simulink model "SimulinkEnv"  (R2024a)
settings: Solver=FixedStepAuto  StartTime=0.0  StopTime=2  RelTol=1e-3
model workspace (MAT data in the model file):
  SL_ROS_VariableLengthArrays_MaxSizes.CommonInfo.ArrayTruncateAction = 'EmitWarning'
  SL_ROS_VariableLengthArrays_MaxSizes.MsgTypeMap = containers.Map
  SL_ROS_VariableLengthArrays_MaxSizes.MsgTypeMap.serialization.keys = {'sensor_msgs/Image'}
  SL_ROS_VariableLengthArrays_MaxSizes.MsgTypeMap.serialization.values{1}(1).PropertyName = 'data'
  SL_ROS_VariableLengthArrays_MaxSizes.MsgTypeMap.serialization.values{1}(1).DataType = 'uint8'
  SL_ROS_VariableLengthArrays_MaxSizes.MsgTypeMap.serialization.values{1}(1).MaxLength = 2764800
  SL_ROS_VariableLengthArrays_MaxSizes.MsgTypeMap.serialization.values{1}(2).PropertyName = 'encoding'
  SL_ROS_VariableLengthArrays_MaxSizes.MsgTypeMap.serialization.values{1}(2).DataType = 'uint8'
  SL_ROS_VariableLengthArrays_MaxSizes.MsgTypeMap.serialization.values{1}(2).MaxLength = 128
  SL_ROS_VariableLengthArrays_MaxSizes.MsgTypeMap.serialization.uniformity = 0
  SL_ROS_VariableLengthArrays_MaxSizes.MsgTypeMap.serialization.keyType = 'char'
  SL_ROS_VariableLengthArrays_MaxSizes.MsgTypeMap.serialization.valueType = 'any'
undefined symbols (not defined in the file): approx_tag_length_cm, Box_pos, BX_x, BX_y, BX_z, coder, home_pos, P_x, P_y, P_z, ros, rTagLocs, Sim3dSensor, SP_pos, stewart_config
libraries: sim3dlib x21, ros2lib x2, sim3dcameralib x2, uavsim3dlib x2, simulink_extras x1, dspvision x1, visionsinks x1, simulink x1
settings Model: PauseTimes=0.5  Creator=dylanfanner  LastModifiedBy=alyss
settings OptimizationCC: EnhancedBackFolding=on  PassReuseOutputArgsAs=Individual arguments  ZeroExternalMemoryAtStartup=off  ZeroInternalMemoryAtStartup=off  MaxStackSize=64  OptimizeBlockOrder=speed  DifferentSizesBufferReuse=on  OptimizationCustomize=off  EfficientTunableParamExpr=on
settings DebuggingCC: ParameterTunabilityLossMsg=error
settings HardwareCC: ProdBitPerLong=64  ProdHWDeviceType=Intel->x86-64 (Linux 64)
settings SFSimCC: MATLABDynamicMemAlloc=off
settings RTWCC: Description=Embedded Coder  SystemTargetFile=ert.tlc  HardwareBoard=Robot Operating System 2 (ROS 2)  TLCOptions="-aInlineSetEventsForThisBaseRateFcn=TLC_FALSE -aSuppressMultiTaskScheduler=TLC_FALSE  -aRateBasedStepFcn=0"  TemplateMakefile=ert_default_tmf  Toolchain=Colcon Tools  TargetLang=C++
settings CodeAppCC: ForceParamTrailComments=on  IgnoreCustomStorageClasses=off  OperatorAnnotations=on  SimulinkDataObjDesc=on  SFDataObjDesc=on  InsertBlockDesc=on
settings ERTTargetCC: CodeInterfacePackaging=C++ class  RootIOFormat=Structure reference

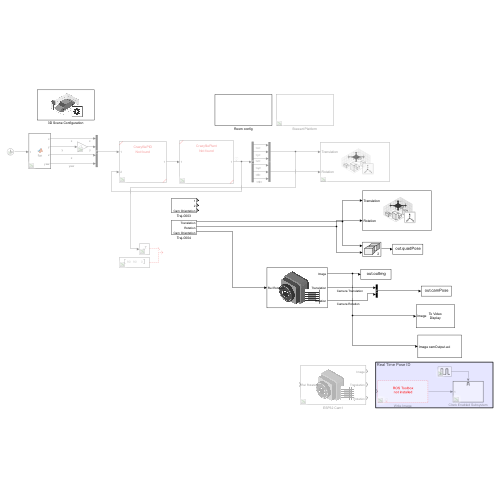
[thumbnail: Simulink's stored preview of the top-level diagram]
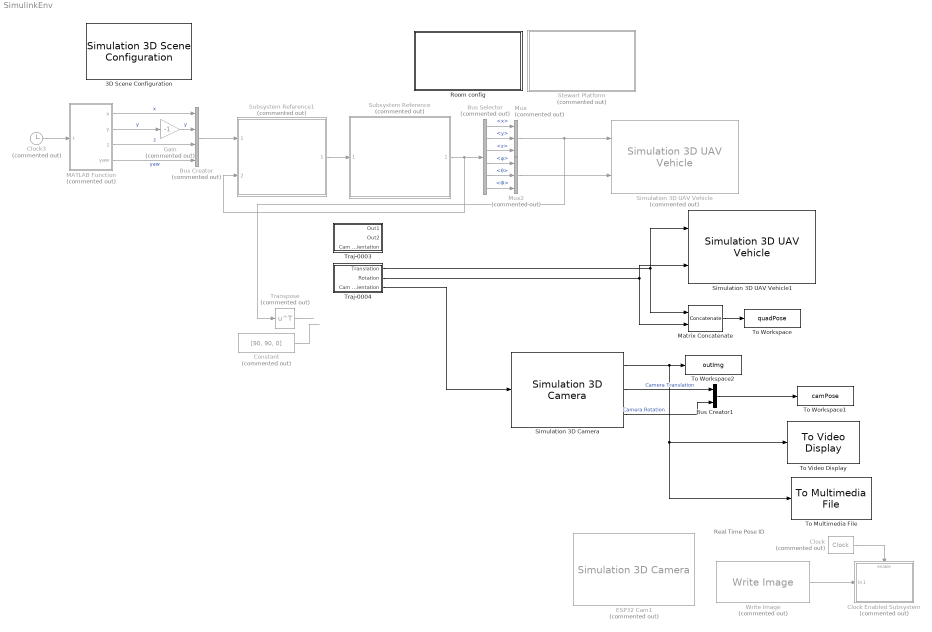
== system SimulinkEnv ==
  note: Real Time Pose ID
  3D Scene Configuration : sim3dlib/Simulation 3D Scene Configuration  Priority=0  ProjectFormat=Default Scenes  SceneDesc=Empty scene  ProjectName=C:\Programs\MATLAB\R2024a\toolbox\shared\sim3d_projects\automotive_project_windows\UE\WindowsNoEditor\VehicleSimulation.exe  ScenePath=/Game/Maps/HwStrght  EnableOpenDRIVE=off  vehTagList={'CrazyFlie';'Custom';'GenericQuad1';'Scene Origin';'Sim3dActor3'}  vehTag=Scene Origin  FreeCameraInitialTranslation=[0, 0, 0]  FreeCameraDefaultInitialTranslation=[-6, 0, 2]  FreeCameraInitialRotation=[0, 0, 0]  FreeCameraDefaultInitialRotation=[0, -15, 0]  OpVisEn=off  Ts=.01  EnableWindow=on  EnableRemoteAccess=off  EnableWeather=off  SunAzimuth=90  SunAltitude=40.0  EnableGeospatialSun=off  Latitude=0  Longitude=0  Date=2023-01-01  Time=10:30:00  GeoTimeZone=-5.0  SunDaylightSaving=off  wind=1  clouds=10  EnableVolumetricClouds=off  CloudCoverage=0  CloudAltitude=6  fog=0  rain=0  RaindropsEffect=off  SnowDensity=0.0  EnableGeospatial=off  UseTrueOrigin=off  OriginHeight=200  OriginLatitude=40.744652  OriginLongitude=-73.988864  MapStyle=Aerial  AdditionalAssetIDs=[]  UseAdvancedSunSky=off  SolarTime=11  TimeZone=-5  Day=21  Month=9  Year=2022  UseDaylightSavingTime=on  DSTStartDay=10  DSTStartMonth=3  DSTEndDay=3  DSTEndMonth=11  DSTSwitchHour=2  sensorTag=MainCamera1  sensorId=1  sensorName=MainCamera1  mountLoc=Origin  offsetFlag=off  tmountOffset=[0, 0, 0]  rmountOffset=[0, 0, 0]  HorizontalResolution=1280  VerticalResolution=720  HorizontalFOV=60  mountPoint=[0 0 0]  mountOrientation=[0 0 0]  aMode=5  ID=1  GeoTrigger=Inactive
      settings: LibrarySourceBlock=sl3dlib/Simulation 3D/Environment/Simulation 3D Scene Configuration
  Bus Creator : BusCreator  Commented=on  Inputs=4
  Bus Creator1 : BusCreator  Inputs=2
  Bus Selector : BusSelector  Commented=on  OutputSignals=Position State.position.x,Position State.position.y,Position State.position.z,Attitude State.attitude.ψ,Attitude State.attitude.θ,Attitude State.attitude.Φ
  Clock : simulink_extras/Flip Flops/Clock  Commented=on  period=0.25
  Clock Enabled Subsystem : Subsystem  Commented=on
  Clock3 : Clock  Commented=on
  Constant : Constant  Commented=on  Value=[90, 90, 0]  VectorParams1D=off
  ESP32 Cam1 : sim3dcameralib/Simulation 3D Camera  Priority=1  Commented=on  sensorTag=Sim3dSensor�  sensorId=3  sensorName=Sim3dSensor�  vehTagList={'CrazyFlie';'Floor';'SPBox';'SPP';'SPapriltexture';'Scene Origin';'Wall1';'Wall2'}  vehTag=CrazyFlie  mountLoc=Origin  offsetFlag=on  tmountOffset=[0, 0, 0]  extTmount=off  rmountOffset=[0, 0, 0]  extRmount=on  FocalLength=cameraParams.FocalLength  OpticalCenter=[640, 360] % I think this is fine  ImageSize=cameraParams.ImageSize  RadialDistortion=cameraParams.RadialDistortion  TangentialDistortion=cameraParams.TangentialDistortion  SensorSkew=0  DepthOutportEnabled=off  SemanticOutportEnabled=off  TransformOutportEnabled=on  SampleTime=-1  mountPoint=[0 0 0]  mountOrientation=[0 0 0]  aMode=6  ID=3
      settings: LibrarySourceBlock=robotsim3dlib/Simulation 3D Camera
  Gain : Gain  Commented=on  Gain=-1
  MATLAB Function : MATLAB Function  Commented=on  TreatAsAtomicUnit=on
  Matrix Concatenate : Concatenate  Mode=Multidimensional array  ConcatenateDimension=2
  Mux : Mux  Commented=on  Inputs=3
  Mux2 : Mux  Commented=on  Inputs=3
  Room config : Subsystem
  Simulation 3D Camera : sim3dcameralib/Simulation 3D Camera  Priority=1  sensorTag=Sim3dSensor�  sensorId=2  sensorName=Sim3dSensor�  vehTagList={'CrazyFlie';'GenericQuad1';'Scene Origin';'Sim3dActor3'}  vehTag=GenericQuad1  mountLoc=Origin  offsetFlag=on  tmountOffset=[0, 0, 0]  extTmount=off  rmountOffset=[0, 0, 0]  extRmount=on  FocalLength=[1107, 1107]  OpticalCenter=[640, 360]  ImageSize=[720, 1280]  RadialDistortion=[0, 0]  TangentialDistortion=[0, 0]  SensorSkew=0  DepthOutportEnabled=off  SemanticOutportEnabled=off  TransformOutportEnabled=on  SampleTime=1/10  mountPoint=[0 0 0]  mountOrientation=[0 0 0]  aMode=6  ID=2
      settings: LibrarySourceBlock=robotsim3dlib/Simulation 3D Camera
  Simulation 3D UAV Vehicle : uavsim3dlib/Simulation 3D UAV Vehicle  Priority=-1  Commented=on  Mesh=Quadrotor  MeshPath=/MathWorksUAVContent/UAVs/HexaRotorUAV/HexaRotor.HexaRotor  Color=Black  ActorName=CrazyFlie  UseGlobalFrame=off  InitialTranslation=[0 0 0]  InitialRotation=[0 0 0]  InitialTranslationGlobal=[0 0 0]  InitialGeoOrigin=[0 0 0]  InitialRotationGlobal=[0 0 0]  SampleTime=-1  ActorType=SimulinkVehicle  ID=C  aMode=4  ActorTag=CrazyFlie
  Simulation 3D UAV Vehicle1 : uavsim3dlib/Simulation 3D UAV Vehicle  Priority=-1  Mesh=Quadrotor  MeshPath=/MathWorksUAVContent/UAVs/HexaRotorUAV/HexaRotor.HexaRotor  Color=Black  ActorName=GenericQuad1  UseGlobalFrame=off  InitialTranslation=[-3 0 1]  InitialRotation=[0 0 0]  InitialTranslationGlobal=[0 0 0]  InitialGeoOrigin=[0 0 0]  InitialRotationGlobal=[0 0 0]  SampleTime=-1  ActorType=SimulinkVehicle  ID=C  aMode=4  ActorTag=GenericQuad1
  Stewart Platform : Subsystem  Commented=on
  Subsystem Reference : Subsystem  Commented=on  ReferencedSubsystem=CrazyfliePlant
  Subsystem Reference1 : Subsystem  Commented=on  ReferencedSubsystem=CrazyfliePID
  To Multimedia File : dspvision/To Multimedia File  outputFilename=camOutput.avi  streamSelection=Video only  videoCompressor=None (uncompressed)  audioCompressor=None (uncompressed)  imagePorts=One multidimensional signal  fileType=AVI  audioDatatype=Determine from input data type  fourcc=RGB  audioBitRate=128  audioQuality=75  videoQuality=75  mj2000CompFactor=10
      settings: LibrarySourceBlock=visionsinks/To Multimedia File
  To Video Display : visionsinks/To Video Display  windowSizeMode=Normal  openAtMdlStart=on  fullScreen=off  videoWindowX=0  videoWindowY=23  saveWindowSize=off  videoWindowWidth=1366  videoWindowHeight=745  inputColorFormat=RGB  inputType=Obsolete  imagePorts=One multidimensional signal  OutputDevice=On-screen video monitor  dataOrg=Column-major  isWindowOpen=off
  To Workspace : ToWorkspace  VariableName=quadPose  SaveFormat=Structure With Time  SampleTime=0.1
  To Workspace1 : ToWorkspace  VariableName=camPose  SaveFormat=Structure With Time  SampleTime=0.1
  To Workspace2 : ToWorkspace  VariableName=outImg  SaveFormat=Structure With Time  SampleTime=0.1
  Traj-0003 : Subsystem
  Traj-0004 : Subsystem
  Transpose : Math  Commented=on  Operator=transpose
  Write Image : ros2lib/Write Image  Commented=on  ImageEncoding=rgb8  EncodingStruct=ros.msg.sensor_msgs.internal.ImageEncoding.info(coder.const('rgb8'))  HasAlpha=off  messageType=sensor_msgs/Image
  wires:
  Subsystem Reference1/1 -> Subsystem Reference/1
  Subsystem Reference/1 -> Subsystem Reference1/2, Bus Selector/1
  Bus Selector/2 -> Mux/2  "<y>"
  Bus Selector/3 -> Mux/3  "<z>"
  Bus Selector/1 -> Mux/1  "<x>"
  Bus Selector/5 -> Mux2/2  "<θ>"
  Bus Selector/4 -> Mux2/1  "<ψ>"
  Bus Selector/6 -> Mux2/3  "<Φ>"
  Bus Creator/1 -> Subsystem Reference1/1
  MATLAB Function/3(z) -> Bus Creator/3  "z"
  MATLAB Function/4(yaw) -> Bus Creator/4  "yaw"
  Mux2/1 -> Simulation 3D UAV Vehicle/2
  Simulation 3D Camera/1 -> To Video Display/1, To Multimedia File/1, To Workspace2/1
  Simulation 3D Camera/3 -> Bus Creator1/2  "Camera Rotation"
  Simulation 3D Camera/2 -> Bus Creator1/1  "Camera Translation"
  Write Image/1 -> Clock Enabled Subsystem/1(In1)
  Clock/1 -> Clock Enabled Subsystem/Enable
  Bus Creator1/1 -> To Workspace1/1
  Gain/1 -> Bus Creator/2  "y"
  Mux/1 -> Simulation 3D UAV Vehicle/1, Transpose/1
  MATLAB Function/1(x) -> Bus Creator/1  "x"
  MATLAB Function/2(y) -> Gain/1  "y"
  Clock3/1 -> MATLAB Function/1(t)
  Constant/1 -> ?
  Transpose/1 -> ?
  Matrix Concatenate/1 -> To Workspace/1
  Traj-0004/1(Translation) -> Simulation 3D UAV Vehicle1/1, Matrix Concatenate/1
  Traj-0004/2(Rotation) -> Simulation 3D UAV Vehicle1/2, Matrix Concatenate/2
  Traj-0004/3(Cam Orientation) -> Simulation 3D Camera/1

== system SimulinkEnv/Clock Enabled Subsystem ==
  In1 : Inport
  Enable : EnablePort
  Publish : ros2lib/Publish  topicSource=Specify your own  topic=/simCam/imgOut  messageType=sensor_msgs/Image  QOSHistory=Keep last  QOSDepth=1  QOSReliability=Reliable  QOSDurability=Volatile  QOSDeadline=Inf  QOSLifespan=Inf  QOSLiveliness=Automatic  QOSLeaseDuration=Inf  QOSAvoidROSNamespaceConventions=off
  wires:
  In1/1 -> Publish/1

== system SimulinkEnv/Room config ==
  Apriltags : sim3dlib/Simulation 3D Actor  Priority=1  ActorName=Sim3dActor1  ParentName=Scene Origin  Operation=Create at setup  InitScriptText=|  SampleTime=-1  Translation=single([0 0 0])  Rotation=single([0 0 0])  Scale=single([1 1 1])  aMode=5  ActorTag=Sim3dActor1  ActorType=Sim3dActor  ID=1
      | % Reserved keywords:
      | % - Actor : handle to this actor object
      | % - World : handle to the world object
      | 
      | % Examples:
      | 
      | % Create a primitive geometry (optional)
      | % Actor.createShape('box', [1 1 1]);
      | 
      | % Initialize values (optional)
      | % Actor.Scale = 1;
      | % Actor.Color = [1 0 0];
  Checkerboards : sim3dlib/Simulation 3D Actor  Priority=1  ActorName=Sim3dActor2  ParentName=Scene Origin  Operation=Create at setup  InitScriptText=|  SampleTime=-1  Translation=single([0 0 0])  Rotation=single([0 0 0])  Scale=single([1 1 1])  aMode=5  ActorTag=Sim3dActor2  ActorType=Sim3dActor  ID=2
      | % Reserved keywords:
      | % - Actor : handle to this actor object
      | % - World : handle to the world object
      | 
      | % Examples:
      | 
      | % Create a primitive geometry (optional)
      | % Actor.createShape('box', [1 1 1]);
      | 
      | % Initialize values (optional)
      | % Actor.Scale = 1;
      | % Actor.Color = [1 0 0];
  Floor : sim3dlib/Simulation 3D Actor  Priority=1  ActorName=Sim3dActor3  ParentName=Scene Origin  Operation=Create at setup  InitScriptText=|  SampleTime=-1  Translation=single([0 0 0])  Rotation=single([0 0 0])  Scale=single([1 1 1])  aMode=5  ActorTag=Sim3dActor3  ActorType=Sim3dActor  ID=3
      | % Reserved keywords:
      | % - Actor : handle to this actor object
      | % - World : handle to the world object
      | 
      | % Examples:
      | 
      | % Create a primitive geometry (optional)
      | % Actor.createShape('box', [1 1 1]);
      | 
      | % Initialize values (optional)
      | % Actor.Scale = 1;
      | % Actor.Color = [1 0 0];
  Walls : sim3dlib/Simulation 3D Actor  Priority=1  ActorName=Sim3dActor4  ParentName=Scene Origin  Operation=Create at setup  InitScriptText=|  SampleTime=-1  Translation=single([0 0 0])  Rotation=single([0 0 0])  Scale=single([1 1 1])  aMode=5  ActorTag=Sim3dActor4  ActorType=Sim3dActor  ID=4
      | % Reserved keywords:
      | % - Actor : handle to this actor object
      | % - World : handle to the world object
      | 
      | % Examples:
      | 
      | % Create a primitive geometry (optional)
      | % Actor.createShape('box', [1 1 1]);
      | 
      | % Initialize values (optional)
      | % Actor.Scale = 1;
      | % Actor.Color = [1 0 0];

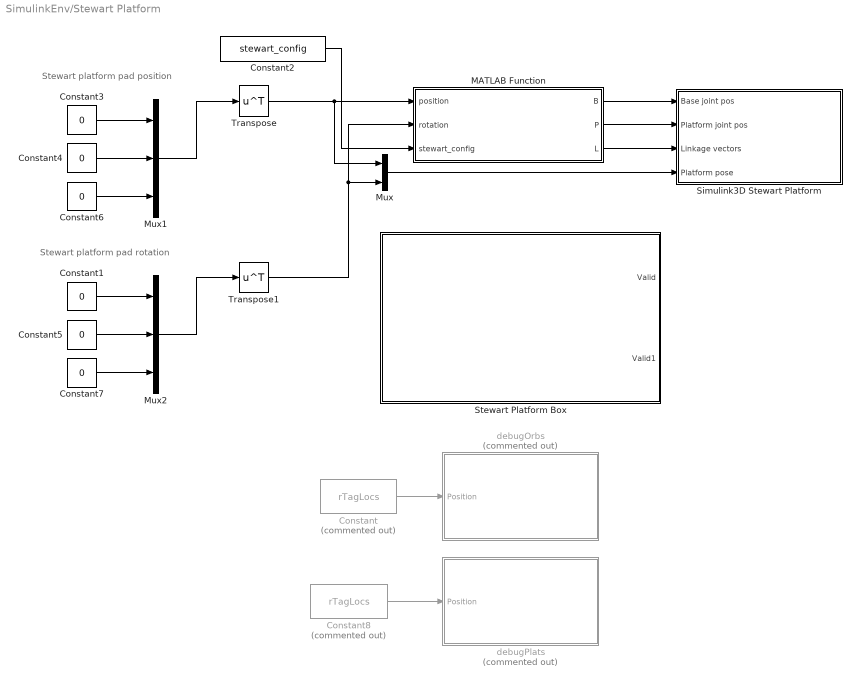
== system SimulinkEnv/Stewart Platform ==
  note: Stewart platform pad rotation
  note: Stewart platform pad position
  Constant : Constant  Commented=on  Value=rTagLocs
  Constant{1,3..7} (6 alike) : Constant  Value=0
  Constant2 : Constant  Value=stewart_config  VectorParams1D=off
  Constant8 : Constant  Commented=on  Value=rTagLocs
  MATLAB Function : MATLAB Function  TreatAsAtomicUnit=on
  Mux : Mux  Inputs=2
  Mux1 : Mux  Inputs=3
  Mux2 : Mux  Inputs=3
  Simulink3D Stewart Platform : Subsystem
  Stewart Platform Box : Subsystem
  Transpose : Math  Operator=transpose
  Transpose1 : Math  Operator=transpose
  debugOrbs : Subsystem  Commented=on  TreatAsAtomicUnit=on
  debugPlats : Subsystem  Commented=on  TreatAsAtomicUnit=on
  wires:
  Mux2/1 -> Transpose1/1
  MATLAB Function/2(P) -> Simulink3D Stewart Platform/2(Platform joint pos)
  Constant3/1 -> Mux1/1
  Constant4/1 -> Mux1/2
  Constant2/1 -> MATLAB Function/3(stewart_config)
  Constant5/1 -> Mux2/2
  Constant1/1 -> Mux2/1
  Mux1/1 -> Transpose/1
  Constant7/1 -> Mux2/3
  Mux/1 -> Simulink3D Stewart Platform/4(Platform pose)
  MATLAB Function/3(L) -> Simulink3D Stewart Platform/3(Linkage vectors)
  Constant6/1 -> Mux1/3
  Transpose1/1 -> MATLAB Function/2(rotation), Mux/2
  MATLAB Function/1(B) -> Simulink3D Stewart Platform/1(Base joint pos)
  Transpose/1 -> MATLAB Function/1(position), Mux/1
  Constant/1 -> debugOrbs/1(Position)
  Constant8/1 -> debugPlats/1(Position)

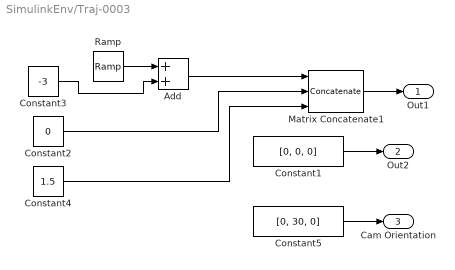
== system SimulinkEnv/Traj-0003 ==
  Add : Sum
  Constant1 : Constant  Value=[0, 0, 0]  VectorParams1D=off
  Constant2 : Constant  Value=0
  Constant3 : Constant  Value=-3
  Constant4 : Constant  Value=1.5
  Constant5 : Constant  Value=[0, 30, 0]  VectorParams1D=off
  Matrix Concatenate1 : Concatenate  NumInputs=3  Mode=Multidimensional array  ConcatenateDimension=2
  Ramp : simulink/Sources/Ramp  slope=0.5  start=0.2  InitialOutput=0
  Out1 : Outport
  Out2 : Outport  Port=2
  Cam Orientation : Outport  Port=3
  wires:
  Constant3/1 -> Add/2
  Ramp/1 -> Add/1
  Matrix Concatenate1/1 -> Out1/1
  Add/1 -> Matrix Concatenate1/1
  Constant1/1 -> Out2/1
  Constant2/1 -> Matrix Concatenate1/2
  Constant4/1 -> Matrix Concatenate1/3
  Constant5/1 -> Cam Orientation/1

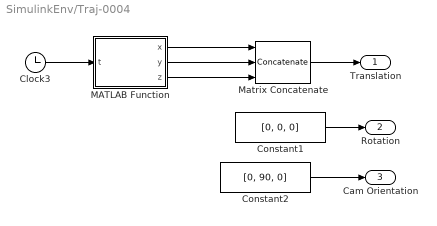
== system SimulinkEnv/Traj-0004 ==
  Clock3 : Clock
  Constant1 : Constant  Value=[0, 0, 0]  VectorParams1D=off
  Constant2 : Constant  Value=[0, 90, 0]  VectorParams1D=off
  MATLAB Function : MATLAB Function  TreatAsAtomicUnit=on
  Matrix Concatenate : Concatenate  NumInputs=3  Mode=Multidimensional array  ConcatenateDimension=2
  Translation : Outport
  Rotation : Outport  Port=2
  Cam Orientation : Outport  Port=3
  wires:
  Clock3/1 -> MATLAB Function/1(t)
  MATLAB Function/2(y) -> Matrix Concatenate/2
  MATLAB Function/3(z) -> Matrix Concatenate/3
  Matrix Concatenate/1 -> Translation/1
  MATLAB Function/1(x) -> Matrix Concatenate/1
  Constant1/1 -> Rotation/1
  Constant2/1 -> Cam Orientation/1

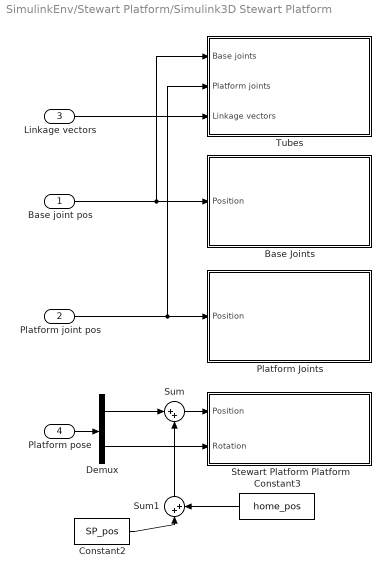
== system SimulinkEnv/Stewart Platform/Simulink3D Stewart Platform ==
  Base joint pos : Inport
  Platform joint pos : Inport  Port=2
  Linkage vectors : Inport  Port=3
  Platform pose : Inport  Port=4
  Base Joints : Subsystem  TreatAsAtomicUnit=on
  Constant2 : Constant  Value=SP_pos  VectorParams1D=off
  Constant3 : Constant  Value=home_pos  VectorParams1D=off
  Demux : Demux  Outputs=2
  Platform Joints : Subsystem  TreatAsAtomicUnit=on
  Stewart Platform Platform : Subsystem
  Sum : Sum  Inputs=|++
  Sum1 : Sum  Inputs=|++
  Tubes : Subsystem  TreatAsAtomicUnit=on
  wires:
  Base joint pos/1 -> Base Joints/1(Position), Tubes/1(Base joints)
  Platform joint pos/1 -> Platform Joints/1(Position), Tubes/2(Platform joints)
  Linkage vectors/1 -> Tubes/3(Linkage vectors)
  Demux/2 -> Stewart Platform Platform/2(Rotation)
  Platform pose/1 -> Demux/1
  Constant3/1 -> Sum1/2
  Constant2/1 -> Sum1/1
  Sum1/1 -> Sum/2
  Sum/1 -> Stewart Platform Platform/1(Position)
  Demux/1 -> Sum/1

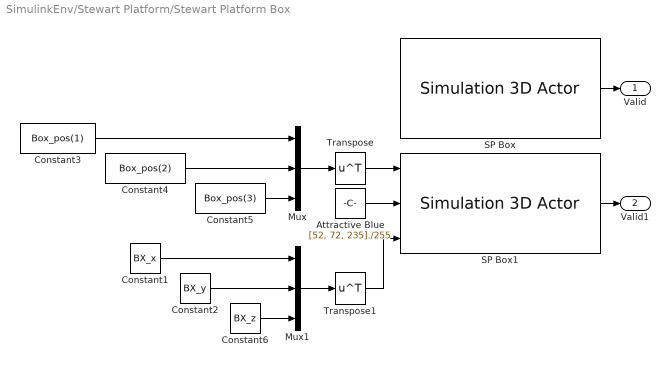
== system SimulinkEnv/Stewart Platform/Stewart Platform Box ==
  Attractive Blue : Constant  Value=[52, 72, 235]./255
  Constant1 : Constant  Value=BX_x
  Constant2 : Constant  Value=BX_y
  Constant3 : Constant  Value=Box_pos(1)
  Constant4 : Constant  Value=Box_pos(2)
  Constant5 : Constant  Value=Box_pos(3)
  Constant6 : Constant  Value=BX_z
  Mux : Mux  Inputs=3
  Mux1 : Mux  Inputs=3
  SP Box : sim3dlib/Simulation 3D Actor  Priority=1  ActorName=SPBox  ParentName=Scene Origin  Operation=Create at setup  InitScriptText=|  SampleTime=-1  Translation=single([0, 0, 0])  Rotation=single([0 0 0])  Scale=single([1 1 1])  aMode=5  ActorTag=SPBox  ActorType=Sim3dActor  ID=C
      | load("roomspec.mat");
      | 
      | Actor.createShape('box', ...
      |                   [1, 1, 1]);
  SP Box1 : sim3dlib/Simulation 3D Actor  Priority=1  ActorName=SPBox  ParentName=Scene Origin  Operation=Reference by name  InitScriptText=|  SampleTime=-1  Translation=single([0, 0, 0])  Rotation=single([0 0 0])  Scale=single([1 1 1])  InputsText=|  aMode=5  ActorTag=Sim3dActor1  ActorType=Sim3dActor  ID=1
      InitScriptText=|
      | load("roomspec.mat");
      | 
      | Actor.createShape('box', ...
      |                   [1, 1, 1]);
      InputsText=|
      | SPBox.Translation
      | SPBox.Color
      | SPBox.Scale
  Transpose : Math  Operator=transpose
  Transpose1 : Math  Operator=transpose
  Valid : Outport
  Valid1 : Outport  Port=2
  wires:
  Transpose1/1 -> SP Box1/3
  Transpose/1 -> SP Box1/1
  Attractive Blue/1 -> SP Box1/2
  Mux1/1 -> Transpose1/1
  Constant6/1 -> Mux1/3
  Constant4/1 -> Mux/2
  Constant2/1 -> Mux1/2
  Mux/1 -> Transpose/1
  SP Box/1 -> Valid/1
  Constant3/1 -> Mux/1
  Constant1/1 -> Mux1/1
  Constant5/1 -> Mux/3
  SP Box1/1 -> Valid1/1

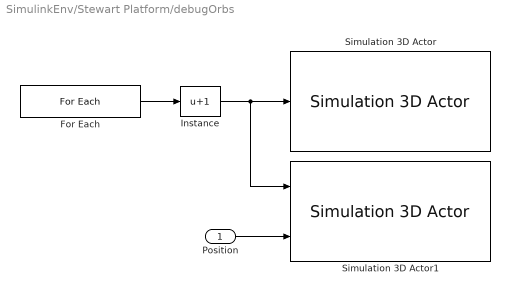
== system SimulinkEnv/Stewart Platform/debugOrbs ==
  Position : Inport  Partition=on  PartitionDimension=1  PartitionWidth=1  PartitionOffset=0
  For Each : ForEach  DisableCoverage=on  ShowIterationIndex=on
  Instance : Bias  Bias=1  SaturateOnIntegerOverflow=off
  Simulation 3D Actor : sim3dlib/Simulation 3D Actor  Priority=1  ActorName=debugOrbs  ParentName=Scene Origin  Operation=Create at step  InitScriptText=|  SampleTime=-1  Translation=single([0 0 0])  Rotation=single([0 0 0])  Scale=single([1 1 1])  aMode=5  ActorTag=Sim3dActor1  ActorType=Sim3dActor  ID=1
      | Actor.createShape('sphere', [0.05, 0.05, 0.05]);
      | Actor.Color = [255, 0, 0]./255;
      | Actor.Shininess = 0;
      | Actor.Metallic = 0;
  Simulation 3D Actor1 : sim3dlib/Simulation 3D Actor  Priority=1  ActorName=debugOrbs  ParentName=Scene Origin  Operation=Reference by instance number  InitScriptText=|  SampleTime=-1  Translation=single([0 0 0])  Rotation=single([0 0 0])  Scale=single([1 1 1])  InputsText=*.Translation  OutputsText=*.Translation  aMode=5  ActorTag=Sim3dActor1  ActorType=Sim3dActor  ID=1
      | Actor.createShape('sphere', [0.05, 0.05, 0.05]);
      | Actor.Color = [125, 125, 125];
  wires:
  For Each/1 -> Instance/1
  Instance/1 -> Simulation 3D Actor/1, Simulation 3D Actor1/1
  Position/1 -> Simulation 3D Actor1/2

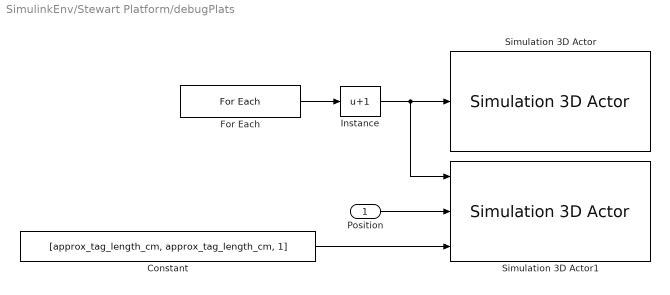
== system SimulinkEnv/Stewart Platform/debugPlats ==
  Position : Inport  Partition=on  PartitionDimension=1  PartitionWidth=1  PartitionOffset=0
  Constant : Constant  Value=[approx_tag_length_cm, approx_tag_length_cm, 1]  VectorParams1D=off
  For Each : ForEach  DisableCoverage=on  ShowIterationIndex=on
  Instance : Bias  Bias=1  SaturateOnIntegerOverflow=off
  Simulation 3D Actor : sim3dlib/Simulation 3D Actor  Priority=1  ActorName=debugPlats  ParentName=Scene Origin  Operation=Create at step  InitScriptText=|  SampleTime=-1  Translation=single([0 0 0])  Rotation=single([0 0 0])  Scale=single([1 1 1])  aMode=5  ActorTag=Sim3dActor1  ActorType=Sim3dActor  ID=1
      | Actor.createShape('plane', [1, 1, 1]);
      | Actor.Color = [125, 125, 125]./255;
      | Actor.Shininess = 0;
      | Actor.Metallic = 0;
  Simulation 3D Actor1 : sim3dlib/Simulation 3D Actor  Priority=1  ActorName=debugPlats  ParentName=Scene Origin  Operation=Reference by instance number  InitScriptText=|  SampleTime=-1  Translation=single([0 0 0])  Rotation=single([0 0 0])  Scale=single([1 1 1])  InputsText=*.Translation *.Scale  OutputsText=*.Translation  aMode=5  ActorTag=Sim3dActor1  ActorType=Sim3dActor  ID=1
      | Actor.createShape('sphere', [0.05, 0.05, 0.05]);
      | Actor.Color = [125, 125, 125];
  wires:
  For Each/1 -> Instance/1
  Instance/1 -> Simulation 3D Actor/1, Simulation 3D Actor1/1
  Position/1 -> Simulation 3D Actor1/2
  Constant/1 -> Simulation 3D Actor1/3

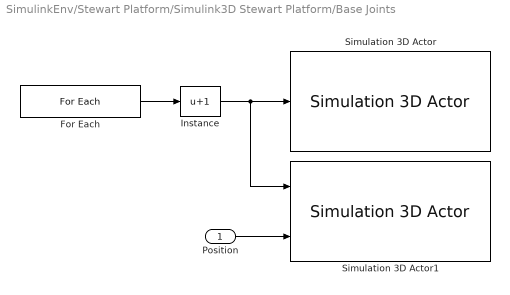
== system SimulinkEnv/Stewart Platform/Simulink3D Stewart Platform/Base Joints ==
  Position : Inport  Partition=on  PartitionDimension=1  PartitionWidth=1  PartitionOffset=0
  For Each : ForEach  DisableCoverage=on  ShowIterationIndex=on
  Instance : Bias  Bias=1  SaturateOnIntegerOverflow=off
  Simulation 3D Actor : sim3dlib/Simulation 3D Actor  Priority=1  ActorName=SPBJ  ParentName=Scene Origin  Operation=Create at step  InitScriptText=|  SampleTime=-1  Translation=single([0 0 0])  Rotation=single([0 0 0])  Scale=single([1 1 1])  aMode=5  ActorTag=Sim3dActor1  ActorType=Sim3dActor  ID=1
      | Actor.createShape('sphere', [0.05, 0.05, 0.05]);
      | Actor.Color = [125, 125, 125]./255;
      | Actor.Shininess = 0;
      | Actor.Metallic = 0;
  Simulation 3D Actor1 : sim3dlib/Simulation 3D Actor  Priority=1  ActorName=SPBJ  ParentName=Scene Origin  Operation=Reference by instance number  InitScriptText=|  SampleTime=-1  Translation=single([0 0 0])  Rotation=single([0 0 0])  Scale=single([1 1 1])  InputsText=*.Translation  OutputsText=*.Translation  aMode=5  ActorTag=Sim3dActor1  ActorType=Sim3dActor  ID=1
      | Actor.createShape('sphere', [0.05, 0.05, 0.05]);
      | Actor.Color = [125, 125, 125];
  wires:
  For Each/1 -> Instance/1
  Instance/1 -> Simulation 3D Actor/1, Simulation 3D Actor1/1
  Position/1 -> Simulation 3D Actor1/2

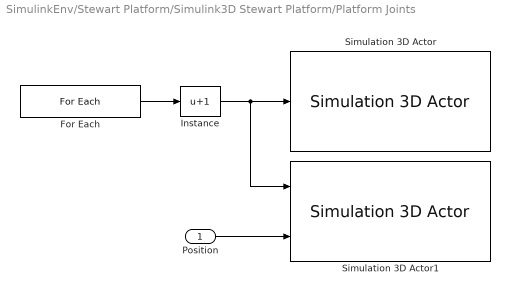
== system SimulinkEnv/Stewart Platform/Simulink3D Stewart Platform/Platform Joints ==
  Position : Inport  Partition=on  PartitionDimension=1  PartitionWidth=1  PartitionOffset=0
  For Each : ForEach  DisableCoverage=on  ShowIterationIndex=on
  Instance : Bias  Bias=1  SaturateOnIntegerOverflow=off
  Simulation 3D Actor : sim3dlib/Simulation 3D Actor  Priority=1  ActorName=SPPJ  ParentName=Scene Origin  Operation=Create at step  InitScriptText=|  SampleTime=-1  Translation=single([0 0 0])  Rotation=single([0 0 0])  Scale=single([1 1 1])  aMode=5  ActorTag=Sim3dActor1  ActorType=Sim3dActor  ID=1
      | Actor.createShape('sphere', [0.015, 0.015, 0.015]);
      | Actor.Color = [125, 125, 125]./255;
      | Actor.Shininess = 0;
      | Actor.Metallic = 0;
  Simulation 3D Actor1 : sim3dlib/Simulation 3D Actor  Priority=1  ActorName=SPPJ  ParentName=Scene Origin  Operation=Reference by instance number  InitScriptText=|  SampleTime=-1  Translation=single([0 0 0])  Rotation=single([0 0 0])  Scale=single([1 1 1])  InputsText=*.Translation  OutputsText=*.Translation  aMode=5  ActorTag=Sim3dActor1  ActorType=Sim3dActor  ID=1
      | Actor.createShape('sphere', [0.05, 0.05, 0.05]);
      | Actor.Color = [125, 125, 125];
  wires:
  For Each/1 -> Instance/1
  Instance/1 -> Simulation 3D Actor/1, Simulation 3D Actor1/1
  Position/1 -> Simulation 3D Actor1/2

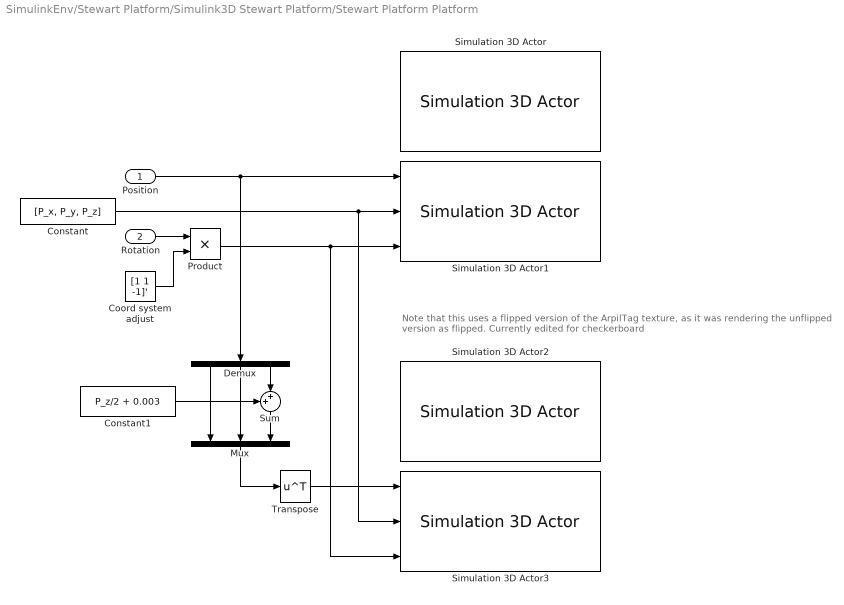
== system SimulinkEnv/Stewart Platform/Simulink3D Stewart Platform/Stewart Platform Platform ==
  note: Note that this uses a flipped version of the ArpilTag texture, as it was rendering the unflipped version as flipped.
      | Currently edited for checkerboard
  Position : Inport
  Rotation : Inport  Port=2
  Constant : Constant  Value=[P_x, P_y, P_z]  VectorParams1D=off
  Constant1 : Constant  Value=P_z/2 + 0.003
  Coord system adjust : Constant  Value=[1 1 -1]'
  Demux : Demux  Outputs=3
  Mux : Mux  Inputs=3
  Product : Product
  Simulation 3D Actor : sim3dlib/Simulation 3D Actor  Priority=1  ActorName=SPP  ParentName=Scene Origin  Operation=Create at setup  InitScriptText=|  SampleTime=-1  Translation=single([0 0 0])  Rotation=single([0 0 0])  Scale=single([1 1 1])  aMode=5  ActorTag=SPP  ActorType=Sim3dActor  ID=C
      | Actor.createShape('box', [1, 1, 1]);
      | Actor.Color = [125, 125, 125]./255;
      | Actor.Shininess = 0;
      | Actor.Metallic = 0;
  Simulation 3D Actor1 : sim3dlib/Simulation 3D Actor  Priority=1  ActorName=SPP  ParentName=Scene Origin  Operation=Reference by name  InitScriptText=|  SampleTime=-1  Translation=single([0 0 0])  Rotation=single([0 0 0])  Scale=single([1 1 1])  InputsText=|  OutputsText=SPP.Translation SPP.Scale  aMode=5  ActorTag=Sim3dActor1  ActorType=Sim3dActor  ID=1
      InitScriptText=|
      | Actor.createShape('sphere', [0.05, 0.05, 0.05]);
      | Actor.Color = [125, 125, 125];
      InputsText=|
      | SPP.Translation
      | SPP.Scale
      | SPP.Rotation
  Simulation 3D Actor2 : sim3dlib/Simulation 3D Actor  Priority=1  ActorName=SPapriltexture  ParentName=Scene Origin  Operation=Create at setup  InitScriptText=|  SampleTime=-1  Translation=single([0 0 0])  Rotation=single([0 0 0])  Scale=single([1 1 1])  aMode=5  ActorTag=SPapriltexture  ActorType=Sim3dActor  ID=C
      | Actor.createShape('plane', [1, 1, 1]);
      | %Actor.Color = [125, 125, 125]./255;
      | Actor.Shininess = 0;
      | Actor.Metallic = 0;
      | Actor.Texture = fullfile(pwd, "Resources/CheckerboardTexture.png");
  Simulation 3D Actor3 : sim3dlib/Simulation 3D Actor  Priority=1  ActorName=SPapriltexture  ParentName=Scene Origin  Operation=Reference by name  InitScriptText=|  SampleTime=-1  Translation=single([0 0 0])  Rotation=single([0 0 0])  Scale=single([1 1 1])  InputsText=|  aMode=5  ActorTag=Sim3dActor1  ActorType=Sim3dActor  ID=1
      InitScriptText=|
      | Actor.createShape('sphere', [0.05, 0.05, 0.05]);
      | Actor.Color = [125, 125, 125];
      InputsText=|
      | SPapriltexture.Translation
      | SPapriltexture.Scale
      | SPapriltexture.Rotation
  Sum : Sum  Inputs=++|
  Transpose : Math  Operator=transpose
  wires:
  Position/1 -> Simulation 3D Actor1/1, Demux/1
  Constant/1 -> Simulation 3D Actor3/2, Simulation 3D Actor1/2
  Rotation/1 -> Product/1
  Product/1 -> Simulation 3D Actor1/3, Simulation 3D Actor3/3
  Coord system adjust/1 -> Product/2
  Demux/1 -> Mux/1
  Demux/2 -> Mux/2
  Demux/3 -> Sum/2
  Sum/1 -> Mux/3
  Constant1/1 -> Sum/1
  Transpose/1 -> Simulation 3D Actor3/1
  Mux/1 -> Transpose/1

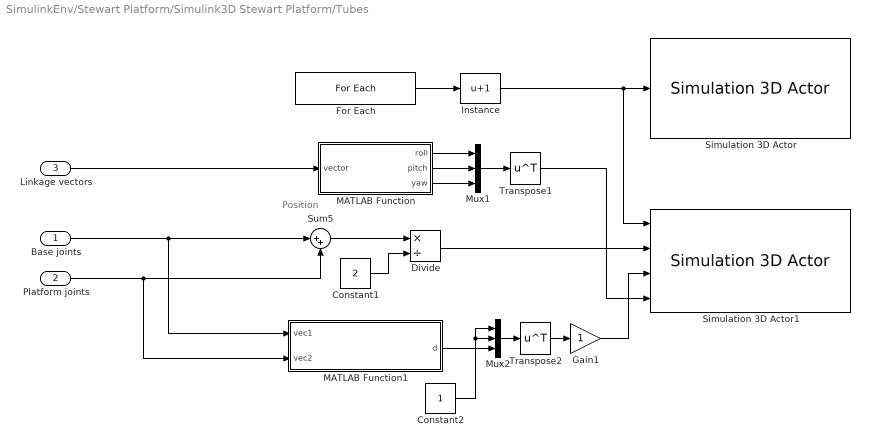
== system SimulinkEnv/Stewart Platform/Simulink3D Stewart Platform/Tubes ==
  note: Position
  Base joints : Inport  Partition=on  PartitionDimension=1  PartitionWidth=1  PartitionOffset=0
  Platform joints : Inport  Port=2  Partition=on  PartitionDimension=1  PartitionWidth=1  PartitionOffset=0
  Linkage vectors : Inport  Port=3  Partition=on  PartitionDimension=1  PartitionWidth=1  PartitionOffset=0
  Constant1 : Constant  Value=2
  Constant2 : Constant
  Divide : Product  Inputs=*/
  For Each : ForEach  DisableCoverage=on  ShowIterationIndex=on
  Gain1 : Gain
  Instance : Bias  Bias=1  SaturateOnIntegerOverflow=off
  MATLAB Function : MATLAB Function  TreatAsAtomicUnit=on
  MATLAB Function1 : MATLAB Function  TreatAsAtomicUnit=on
  Mux1 : Mux  Inputs=3
  Mux2 : Mux  Inputs=3
  Simulation 3D Actor : sim3dlib/Simulation 3D Actor  Priority=1  ActorName=SPlinkages  ParentName=Scene Origin  Operation=Create at step  InitScriptText=|  SampleTime=-1  Translation=single([0 0 0])  Rotation=single([0 0 0])  Scale=single([1 1 1])  aMode=5  ActorTag=Sim3dActor1  ActorType=Sim3dActor  ID=1
      | Actor.createShape('tube', [0.01, 0.01, 1], 0.75, 10, 3);
      | Actor.Color = [60, 60, 60]./255;
      | Actor.Shininess = 0;
      | Actor.Metallic = 0;
  Simulation 3D Actor1 : sim3dlib/Simulation 3D Actor  Priority=1  ActorName=SPlinkages  ParentName=Scene Origin  Operation=Reference by instance number  InitScriptText=|  SampleTime=-1  Translation=single([0 0 0])  Rotation=single([0 0 0])  Scale=single([1 1 1])  InputsText=|  OutputsText=*.Translation  aMode=5  ActorTag=Sim3dActor1  ActorType=Sim3dActor  ID=1
      InitScriptText=|
      | Actor.createShape('sphere', [0.05, 0.05, 0.05]);
      | Actor.Color = [125, 125, 125];
      InputsText=|
      | *.Translation
      | *.Scale
      | *.Rotation
  Sum5 : Sum  Inputs=|++
  Transpose1 : Math  Operator=transpose
  Transpose2 : Math  Operator=transpose
  wires:
  For Each/1 -> Instance/1
  Instance/1 -> Simulation 3D Actor/1, Simulation 3D Actor1/1
  Base joints/1 -> MATLAB Function1/1(vec1), Sum5/1
  Platform joints/1 -> MATLAB Function1/2(vec2), Sum5/2
  Sum5/1 -> Divide/1
  Constant1/1 -> Divide/2
  Divide/1 -> Simulation 3D Actor1/2
  Linkage vectors/1 -> MATLAB Function/1(vector)
  Mux1/1 -> Transpose1/1
  MATLAB Function/1(roll) -> Mux1/1
  MATLAB Function/2(pitch) -> Mux1/2
  Transpose1/1 -> Simulation 3D Actor1/4
  MATLAB Function/3(yaw) -> Mux1/3
  Transpose2/1 -> Gain1/1
  Mux2/1 -> Transpose2/1
  Constant2/1 -> Mux2/1, Mux2/2
  MATLAB Function1/1(d) -> Mux2/3
  Gain1/1 -> Simulation 3D Actor1/3

== matlab function SimulinkEnv/Stewart Platform/Simulink3D Stewart Platform/Tubes/MATLAB Function1 ==
  data: vec1 input; d output; vec2 input
function d = euclid_dist(vec1, vec2)

d = sqrt(sum((vec1 - vec2).^2));

== matlab function SimulinkEnv/Stewart Platform/Simulink3D Stewart Platform/Tubes/MATLAB Function ==
  data: vector input; roll output; pitch output; yaw output
function [roll, pitch, yaw] = vec_to_deg(vector)

pitch = atan2(sqrt(vector(1)^2 + vector(2)^2), vector(3));
roll = 0;
yaw = pi/2 + pi - atan2(vector(1),vector(2));

== matlab function SimulinkEnv/Stewart Platform/MATLAB Function ==
  data: position input; B output; rotation input; stewart_config input; P output; L output
function [B, P, L] = call_stewart(position, rotation, stewart_config)

[B,P,L] = stewart(position, rotation, stewart_config);

== matlab function SimulinkEnv/Traj-0004/MATLAB Function ==
  data: x output; t input; y output; z output
function [x, y, z] = fcn(t)

    
    x = 0;
    y = 0;
    z = (1.5/2)*t;
    
    if t>=2
        x =0;
        y=(0.2/2)*t;
        z=1.5;
    end
    
    if t>=4
        x =0;
        y=0.1*(-t+6);
        z=(0.3/2)*t+0.9;
    end
    
    if t>=6
        x =0;
        y=0.1*(-t+6);
        z=1.8;
    end
    
    if t>=8
        x=0;
        y=0.1*(t-10);
        z=(-0.15*t)+3;
    end

end

== matlab function SimulinkEnv/MATLAB Function ==
  data: x output; t input; y output; z output; yaw output
function [x, y, z, yaw] = fcn(t)
x = 0;
y = 0;
z = 1;
yaw = 0;

if t>2
    x =0.2;
    y=0;
    z=1;
end

if t>4
    x =0;
    y=0;
    z=1.5;
end

if t>6
    x =-0.2;
    y=0;
    z=1.5;
end

if t>8
    x=0;
    y=0;
    z=1;
end


if (t<9)
    yaw = 0;
elseif (t>9)
    yaw = (t-9)/6 * 45;
end
